simulink model "CopyZeroMain"  (R2023b)
settings: Solver=VariableStepAuto  StartTime=0.0  StopTime=10.0  RelTol=1e-3
values from neighbouring files (symbols this model uses):
  a1 = 40    [FK.m]    (also in IK_Analytical.m = 0.04; IK_MDH.m = 0.04; IK_Position.m = 0.04; IK_Solver.m = 0.04)
  a2 = 275    [FK.m]    (also in IK_Analytical.m = 0.275; IK_MDH.m = 0.275; IK_Position.m = 0.275; IK_Solver.m = 0.275)
  a3 = 25    [FK.m]    (also in IK_Analytical.m = 0.025; IK_MDH.m = 0.025; IK_Position.m = 0.025; IK_Solver.m = 0.025)
  d1 = 342    [FK.m]    (also in IK_Analytical.m = 0.342; IK_MDH.m = 0.342; IK_Position.m = 0.342; IK_Solver.m = 0.342)
  d4 = 280    [FK.m]    (also in IK_Analytical.m = 0.28; IK_MDH.m = 0.28; IK_Position.m = 0.28; IK_Solver.m = 0.28)
  D_H = [ ... (first row only)    [set_mode_parameter.m]
  Ic111 = 0    [set_mode_parameter.m]
  Ic112 = 0    [set_mode_parameter.m]
  Ic113 = 0    [set_mode_parameter.m]
  Ic122 = 0    [set_mode_parameter.m]
  Ic123 = 0    [set_mode_parameter.m]
  Ic133 = 1.3676    [set_mode_parameter.m]
  Ic211 = 8.8194    [set_mode_parameter.m]
  Ic212 = 0    [set_mode_parameter.m]
  Ic213 = 0    [set_mode_parameter.m]
  Ic222 = 6.0549    [set_mode_parameter.m]
  Ic223 = 0    [set_mode_parameter.m]
  Ic233 = 0.9569    [set_mode_parameter.m]
  Ic311 = 0.0332    [set_mode_parameter.m]
  Ic312 = 0    [set_mode_parameter.m]
  Ic313 = 0    [set_mode_parameter.m]
  Ic322 = 1.8442    [set_mode_parameter.m]
  Ic323 = 0    [set_mode_parameter.m]
  Ic333 = 1.0560    (= 1.056)    [set_mode_parameter.m]
  Ic411 = 0.1448    [set_mode_parameter.m]
  Ic412 = 0    [set_mode_parameter.m]
  Ic413 = 0    [set_mode_parameter.m]
  Ic422 = 0.0015    [set_mode_parameter.m]
  Ic423 = 0    [set_mode_parameter.m]
  Ic433 = 0.0822    [set_mode_parameter.m]
  Ic511 = 0    [set_mode_parameter.m]
  Ic512 = 0    [set_mode_parameter.m]
  Ic513 = 0    [set_mode_parameter.m]
  Ic522 = 0.0121    [set_mode_parameter.m]
  Ic523 = 0    [set_mode_parameter.m]
  Ic533 = 0.0299    [set_mode_parameter.m]
  Ic611 = 0.0134    [set_mode_parameter.m]
  Ic612 = 0    [set_mode_parameter.m]
  Ic613 = 0    [set_mode_parameter.m]
  Ic622 = 0    [set_mode_parameter.m]
  Ic623 = 0    [set_mode_parameter.m]
  Ic633 = 0.0051    [set_mode_parameter.m]
  m = (c1*px + s1*py) - dt*(c1*ax + s1*ay) - a1    [IK_6DOF_Robot.m]    (also in IK_MDH.m = pwx_1 - a1; IK_MDH_Robot.m = rho - a1)
  m1 = 0.167    [set_mode_parameter.m]
  m2 = 1    [set_mode_parameter.m]
  m3 = 0.5    [set_mode_parameter.m]
  m4 = 0.333    [set_mode_parameter.m]
  m5 = 0.25    [set_mode_parameter.m]
  m6 = 0.2    [set_mode_parameter.m]
  mc11 = 0    [set_mode_parameter.m]
  mc12 = 0    [set_mode_parameter.m]
  mc13 = 0.2    [set_mode_parameter.m]
  mc21 = 0.1291    [set_mode_parameter.m]
  mc22 = 0    [set_mode_parameter.m]
  mc23 = 3.3117    [set_mode_parameter.m]
  mc31 = 1.6484    [set_mode_parameter.m]
  mc32 = 0    [set_mode_parameter.m]
  mc33 = 0.8748    [set_mode_parameter.m]
  mc41 = 0.3200    (= 0.32)    [set_mode_parameter.m]
  mc42 = 0.2324    [set_mode_parameter.m]
  mc43 = 0.7083    [set_mode_parameter.m]
  mc51 = 0.4574    [set_mode_parameter.m]
  mc52 = 0    [set_mode_parameter.m]
  mc53 = 0.6427    [set_mode_parameter.m]
  mc61 = 0.3200    (= 0.32)    [set_mode_parameter.m]
  mc62 = -0.0513    [set_mode_parameter.m]
  mc63 = 0.6417    [set_mode_parameter.m]
  N = size(waypoints, 2)    [run_trajectory.m]
  s = zc - d(1)    [inverse_kinematics_6dof.m]
  XB4 = SerialLink([L1 L2 L3 L4 L5 L6], 'name', 'XB4')    [Toolbox_Motheds_1.m]
undefined symbols (not defined in the file or in its folder): X, Y, Z
libraries: sm_lib x57, nesl_utility x11
(part 2 of 2)

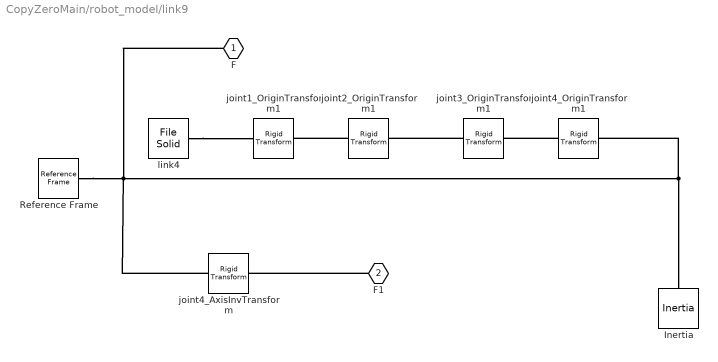
== system CopyZeroMain/robot_model/link9 ==
  Inertia : sm_lib/Body Elements/Inertia  InertiaType=Custom  Mass=m4  MassUnits=kg  CenterOfMass=[mc41 mc42 mc43]  CenterOfMassUnits=m  MomentsOfInertia=[Ic411 Ic422 Ic433]  MomentsOfInertiaUnits=kg*m^2  ProductsOfInertia=[Ic423 Ic413 Ic412]  ProductsOfInertiaUnits=kg*m^2  GraphicType=Marker  MarkerShape=Inertia  MarkerSize=20  GraphicVisPropType=SimpleVisualProperties  GraphicDiffuseColor=[0.5 0.5 0.5]  GraphicSpecularColor=[0.5 0.5 0.5 1.0]  GraphicAmbientColor=[0.15 0.15 0.15 1.0]  GraphicEmissiveColor=[0.0 0.0 0.0 1.0]  GraphicShininess=75  GraphicOpacity=1.0
  Reference Frame : sm_lib/Frames and Transforms/Reference Frame
  joint1_OriginTransform1 : sm_lib/Frames and Transforms/Rigid Transform  TranslationMethod=Cartesian  TranslationStandardOffset=0  TranslationStandardOffsetUnits=m  TranslationStandardAxis=+Z  TranslationCartesianOffset=[0 0 d1]  TranslationCartesianOffsetUnits=m  TranslationROffset=0  TranslationROffsetUnits=m  TranslationZOffset=0  TranslationZOffsetUnits=m  TranslationThetaOffset=0  TranslationThetaOffsetUnits=deg  RotationMethod=RotationSequence  RotationAngleUnits=deg  RotationStandardAxis=+Z  RotationAngle=0.0  RotationArbitraryAxis=[0 0 1]  FollAlignAxisA=+X  BaseAlignAxisA=+Y  FollAlignAxisB=+Y  BaseAlignAxisB=+Z  RotationSequenceAxes=BaseAxes  RotationSequence=XYZ  RotationSequenceAngles=[0 0 0]  RotationSequenceAnglesUnits=rad  RotationMatrix=[1 0 0; 0 1 0; 0 0 1]  Quaternion=[1 0 0 0]
  joint2_OriginTransform1 : sm_lib/Frames and Transforms/Rigid Transform  TranslationMethod=Cartesian  TranslationStandardOffset=0  TranslationStandardOffsetUnits=m  TranslationStandardAxis=+Z  TranslationCartesianOffset=[a1 0 0]  TranslationCartesianOffsetUnits=m  TranslationROffset=0  TranslationROffsetUnits=m  TranslationZOffset=0  TranslationZOffsetUnits=m  TranslationThetaOffset=0  TranslationThetaOffsetUnits=deg  RotationMethod=RotationSequence  RotationAngleUnits=deg  RotationStandardAxis=+Z  RotationAngle=0.0  RotationArbitraryAxis=[0 0 1]  FollAlignAxisA=+X  BaseAlignAxisA=+Y  FollAlignAxisB=+Y  BaseAlignAxisB=+Z  RotationSequenceAxes=FollowerAxes  RotationSequence=XYZ  RotationSequenceAngles=[-pi/2 0 -pi/2]  RotationSequenceAnglesUnits=rad  RotationMatrix=[1 0 0; 0 1 0; 0 0 1]  Quaternion=[1 0 0 0]
  joint3_OriginTransform1 : sm_lib/Frames and Transforms/Rigid Transform  TranslationMethod=Cartesian  TranslationStandardOffset=0  TranslationStandardOffsetUnits=m  TranslationStandardAxis=+Z  TranslationCartesianOffset=[a2 0 0]  TranslationCartesianOffsetUnits=m  TranslationROffset=0  TranslationROffsetUnits=m  TranslationZOffset=0  TranslationZOffsetUnits=m  TranslationThetaOffset=0  TranslationThetaOffsetUnits=deg  RotationMethod=RotationSequence  RotationAngleUnits=deg  RotationStandardAxis=+Z  RotationAngle=0.0  RotationArbitraryAxis=[0 0 1]  FollAlignAxisA=+X  BaseAlignAxisA=+Y  FollAlignAxisB=+Y  BaseAlignAxisB=+Z  RotationSequenceAxes=FollowerAxes  RotationSequence=XYZ  RotationSequenceAngles=[0 0 0]  RotationSequenceAnglesUnits=rad  RotationMatrix=[1 0 0; 0 1 0; 0 0 1]  Quaternion=[1 0 0 0]
  joint4_AxisInvTransform : sm_lib/Frames and Transforms/Rigid Transform  TranslationMethod=Cartesian  TranslationStandardOffset=0  TranslationStandardOffsetUnits=m  TranslationStandardAxis=+Z  TranslationCartesianOffset=[0 0 0]  TranslationCartesianOffsetUnits=m  TranslationROffset=0  TranslationROffsetUnits=m  TranslationZOffset=0  TranslationZOffsetUnits=m  TranslationThetaOffset=0  TranslationThetaOffsetUnits=deg  RotationMethod=RotationSequence  RotationAngleUnits=rad  RotationStandardAxis=+Z  RotationAngle=1.570796  RotationArbitraryAxis=[0 1 0]  FollAlignAxisA=+X  BaseAlignAxisA=+Y  FollAlignAxisB=+Y  BaseAlignAxisB=+Z  RotationSequenceAxes=FollowerAxes  RotationSequence=XYZ  RotationSequenceAngles=[pi/2 0 0]  RotationSequenceAnglesUnits=rad  RotationMatrix=[1 0 0; 0 1 0; 0 0 1]  Quaternion=[1 0 0 0]
  joint4_OriginTransform1 : sm_lib/Frames and Transforms/Rigid Transform  TranslationMethod=Cartesian  TranslationStandardOffset=0  TranslationStandardOffsetUnits=m  TranslationStandardAxis=+Z  TranslationCartesianOffset=[a3 d4 0]  TranslationCartesianOffsetUnits=m  TranslationROffset=0  TranslationROffsetUnits=m  TranslationZOffset=0  TranslationZOffsetUnits=m  TranslationThetaOffset=0  TranslationThetaOffsetUnits=deg  RotationMethod=RotationSequence  RotationAngleUnits=deg  RotationStandardAxis=+Z  RotationAngle=0.0  RotationArbitraryAxis=[0 0 1]  FollAlignAxisA=+X  BaseAlignAxisA=+Y  FollAlignAxisB=+Y  BaseAlignAxisB=+Z  RotationSequenceAxes=FollowerAxes  RotationSequence=XYZ  RotationSequenceAngles=[-pi/2 0 0]  RotationSequenceAnglesUnits=rad  RotationMatrix=[1 0 0; 0 1 0; 0 0 1]  Quaternion=[1 0 0 0]
  link4 : sm_lib/Body Elements/File Solid  ExtGeomFileName=/home/jiehuang/Documents/Custom-Robot/Matlab_Study/Matlab2023Project/IntroductionBook/程序/XB4模型/XB4-4.STL  UnitType=Custom  ExtGeomFileUnits=mm  StepReaderType=HEX  ExportConvexHullGeometry=off  InertiaType=Custom  Mass=0  MassUnits=kg  CenterOfMass=[0 0 0]  CenterOfMassUnits=m  MomentsOfInertia=[0 0 0]  MomentsOfInertiaUnits=kg*m^2  ProductsOfInertia=[0 0 0]  ProductsOfInertiaUnits=kg*m^2  BasedOnType=Density  Density=1000  DensityUnits=kg/(m^3)  DoExposeReferenceFrame=on  SerializedFrames=<Frames/>  GraphicType=FromGeometry  MarkerShape=Sphere  MarkerSize=10  GraphicVisPropType=SimpleVisualProperties  GraphicDiffuseColor=[0.5 0.5 0.5]  GraphicSpecularColor=[0.5 0.5 0.5 1.0]  GraphicAmbientColor=[0.15 0.15 0.15 1.0]  GraphicEmissiveColor=[0.0 0.0 0.0 1.0]  GraphicShininess=75  GraphicOpacity=1.0
  F : PMIOPort  Side=Left
  F1 : PMIOPort  Port=2  Side=Right
  connections:
  Reference Frame/RConn1 -- Inertia/RConn1 -- joint4_OriginTransform1/RConn1 -- F/RConn1 -- joint4_AxisInvTransform/LConn1
  F1/RConn1 -- joint4_AxisInvTransform/RConn1
  joint4_OriginTransform1/LConn1 -- joint3_OriginTransform1/RConn1
  joint3_OriginTransform1/LConn1 -- joint2_OriginTransform1/RConn1
  joint2_OriginTransform1/LConn1 -- joint1_OriginTransform1/RConn1
  link4/RConn1 -- joint1_OriginTransform1/LConn1

== matlab function CopyZeroMain/MATLAB Function1 ==
  data: thetas input; theta output; index input
function theta = theta_selection(thetas, index)

theta = thetas(index, :);

== matlab function CopyZeroMain/inv_kinematic/MATLAB Function13 ==
  data: joint_thetas input; thetas_ret output
function thetas_ret = joint_rad2deg(joint_thetas)
thetas_ret = joint_thetas;
for i = 1:4
    for j = 1:6
        thetas_ret(i,j) = rad2deg(thetas_ret(i,j));
    end
end

== matlab function CopyZeroMain/inv_kinematic/MATLAB Function1 ==
  data: T_target input; joint_thetas_ret output; joint_thetas input; D_H input
function joint_thetas_ret  = get_theta2(T_target, joint_thetas, D_H)
joint_thetas_ret = zeros(4,6);
joint_thetas_ret(1,:) = joint_thetas(1,:);
joint_thetas_ret(2,:) = joint_thetas(1,:);
joint_thetas_ret(3,:) = joint_thetas(2,:);
joint_thetas_ret(4,:) = joint_thetas(2,:);
joint_thetas_ret(1,2) = get_theta2_1(T_target, joint_thetas_ret(1,3), D_H);
joint_thetas_ret(2,2) = get_theta2_2(T_target, joint_thetas_ret(2,3), D_H);
joint_thetas_ret(3,2) = get_theta2_1(T_target, joint_thetas_ret(3,3), D_H);
joint_thetas_ret(4,2) = get_theta2_2(T_target, joint_thetas_ret(4,3), D_H);
end

function theta2_1 = get_theta2_1(T_target, theta3, D_H)
a_cow = D_H(:, 1);
d_cow = D_H(:, 3);
a2 = a_cow(3);
a3 = a_cow(4);
d4 = d_cow(4);
pz = T_target(3,4);
u1_theta2 = -(a2 + (a2^2 + 2*cos(theta3)*a2*a3 - 2*sin(theta3)*a2*d4 + a3^2 + d4^2 - pz^2)^(1/2) + a3*cos(theta3) - d4*sin(theta3))/(d4*cos(theta3) - pz + a3*sin(theta3));
theta2_1 = atan(u1_theta2)*2;
end

function theta2_2 = get_theta2_2(T_target, theta3, D_H)
a_cow = D_H(:, 1);
d_cow = D_H(:, 3);
a2 = a_cow(3);
a3 = a_cow(4);
d4 = d_cow(4);
pz = T_target(3,4);
u2_theta2 = -(a2 - (a2^2 + 2*cos(theta3)*a2*a3 - 2*sin(theta3)*a2*d4 + a3^2 + d4^2 - pz^2)^(1/2) + a3*cos(theta3) - d4*sin(theta3))/(d4*cos(theta3) - pz + a3*sin(theta3));
theta2_2 = atan(u2_theta2)*2;
end

== matlab function CopyZeroMain/inv_kinematic/MATLAB Function ==
  data: T_target input; joint_theatas_ret output; D_H input
function joint_theatas_ret  = get_theta3(T_target, D_H)
a_cow = D_H(:, 1);
d_cow = D_H(:, 3);
a2 = a_cow(3);
a3 = a_cow(4);
d4 = d_cow(4);
px = T_target(1,4);
py = T_target(2,4);
pz = T_target(3,4);
joint_theatas_ret = zeros(2,6);

u1_theta3 = -(2*a2*d4 + (- a2^4 + 2*a2^2*a3^2 + 2*a2^2*d4^2 + 2*a2^2*px^2 + 2*a2^2*py^2 + 2*a2^2*pz^2 - a3^4 - 2*a3^2*d4^2 + 2*a3^2*px^2 + 2*a3^2*py^2 + 2*a3^2*pz^2 - d4^4 + 2*d4^2*px^2 + 2*d4^2*py^2 + 2*d4^2*pz^2 - px^4 - 2*px^2*py^2 - 2*px^2*pz^2 - py^4 - 2*py^2*pz^2 - pz^4)^(1/2))/(- a2^2 + 2*a2*a3 - a3^2 - d4^2 + px^2 + py^2 + pz^2);
u2_theta3 = -(2*a2*d4 - (- a2^4 + 2*a2^2*a3^2 + 2*a2^2*d4^2 + 2*a2^2*px^2 + 2*a2^2*py^2 + 2*a2^2*pz^2 - a3^4 - 2*a3^2*d4^2 + 2*a3^2*px^2 + 2*a3^2*py^2 + 2*a3^2*pz^2 - d4^4 + 2*d4^2*px^2 + 2*d4^2*py^2 + 2*d4^2*pz^2 - px^4 - 2*px^2*py^2 - 2*px^2*pz^2 - py^4 - 2*py^2*pz^2 - pz^4)^(1/2))/(- a2^2 + 2*a2*a3 - a3^2 - d4^2 + px^2 + py^2 + pz^2);
theta3_1 = atan(u1_theta3)*2;
theta3_2 = atan(u2_theta3)*2;
joint_theatas_ret(1, 3) = theta3_1;
joint_theatas_ret(2, 3) = theta3_2;
end

== matlab function CopyZeroMain/inv_kinematic/MATLAB Function2 ==
  data: T_target input; joint_thetas output; joint_thetas input; D_H input
function joint_thetas  = get_theta1(T_target, joint_thetas, D_H)
joint_thetas(1,1) = get_theta1_(T_target, joint_thetas(1,:), D_H);
joint_thetas(2,1) = get_theta1_(T_target, joint_thetas(2,:), D_H);
joint_thetas(3,1) = get_theta1_(T_target, joint_thetas(3,:), D_H);
joint_thetas(4,1) = get_theta1_(T_target, joint_thetas(4,:), D_H);
end

function theta1_1 = get_theta1_(T_target, thetas, D_H)
a_cow = D_H(:, 1);
d_cow = D_H(:, 3);
a2 = a_cow(3);
a3 = a_cow(4);
d4 = d_cow(4);
px = T_target(1,4);
py = T_target(2,4);
pz = T_target(3,4);

theta2 = thetas(2);
theta3 = thetas(3);

v1 = (cos(theta2)*(a2 + a3*cos(theta3) - d4*sin(theta3)) + sin(theta2)*(d4*cos(theta3) + a3*sin(theta3)));
v2 = -px/v1;

% 设置容忍度
tolerance = 1e-4;

u1_theta1 = ((v2+1)/(1-v2))^(1/2);
if abs(py - (2*u1_theta1*v1)/(u1_theta1^2 + 1)) > tolerance
    u1_theta1 = -u1_theta1;
end
theta1_1 = atan(u1_theta1)*2;
end

== matlab function CopyZeroMain/inv_kinematic/MATLAB Function3 ==
  data: T_target input; joint_thetas_ret output; joint_thetas input; D_H input
function joint_thetas_ret  = get_theta5(T_target, joint_thetas, D_H)
joint_thetas_ret = joint_thetas;
for i = 1:4
    joint_thetas_ret(i, 5) = get_theta5_(T_target, joint_thetas_ret(i, :), D_H);
end
end

function theta5 = get_theta5_(T_target, thetas, D_H)
a_cow = D_H(:, 1);
d_cow = D_H(:, 3);
a2 = a_cow(3);
a3 = a_cow(4);
d4 = d_cow(4);
px = T_target(1,4);
py = T_target(2,4);
pz = T_target(3,4);
nx = T_target(1,1);
ny = T_target(2,1);
nz = T_target(3,1);
ox = T_target(1,2);
oy = T_target(2,2);
oz = T_target(3,2);
ax= T_target(1,3);
ay= T_target(2,3);
az= T_target(3,3);
theta2 = thetas(2);
theta3 = thetas(3);
theta1 = thetas(1);

r32 = - (oz*(cos(theta2)*cos(theta3) + sin(theta2)*sin(theta3)))/(cos(theta2)^2*cos(theta3)^2 + cos(theta2)^2*sin(theta3)^2 + cos(theta3)^2*sin(theta2)^2 + sin(theta2)^2*sin(theta3)^2) - (ox*(cos(theta1)*cos(theta2)*sin(theta3) - cos(theta1)*cos(theta3)*sin(theta2)))/(cos(theta1)^2*cos(theta2)^2*cos(theta3)^2 + cos(theta1)^2*cos(theta2)^2*sin(theta3)^2 + cos(theta1)^2*cos(theta3)^2*sin(theta2)^2 + cos(theta1)^2*sin(theta2)^2*sin(theta3)^2 + cos(theta2)^2*cos(theta3)^2*sin(theta1)^2 + cos(theta2)^2*sin(theta1)^2*sin(theta3)^2 + cos(theta3)^2*sin(theta1)^2*sin(theta2)^2 + sin(theta1)^2*sin(theta2)^2*sin(theta3)^2) - (oy*(cos(theta2)*sin(theta1)*sin(theta3) - cos(theta3)*sin(theta1)*sin(theta2)))/(cos(theta1)^2*cos(theta2)^2*cos(theta3)^2 + cos(theta1)^2*cos(theta2)^2*sin(theta3)^2 + cos(theta1)^2*cos(theta3)^2*sin(theta2)^2 + cos(theta1)^2*sin(theta2)^2*sin(theta3)^2 + cos(theta2)^2*cos(theta3)^2*sin(theta1)^2 + cos(theta2)^2*sin(theta1)^2*sin(theta3)^2 + cos(theta3)^2*sin(theta1)^2*sin(theta2)^2 + sin(theta1)^2*sin(theta2)^2*sin(theta3)^2);
r31 = - (nz*(cos(theta2)*cos(theta3) + sin(theta2)*sin(theta3)))/(cos(theta2)^2*cos(theta3)^2 + cos(theta2)^2*sin(theta3)^2 + cos(theta3)^2*sin(theta2)^2 + sin(theta2)^2*sin(theta3)^2) - (nx*(cos(theta1)*cos(theta2)*sin(theta3) - cos(theta1)*cos(theta3)*sin(theta2)))/(cos(theta1)^2*cos(theta2)^2*cos(theta3)^2 + cos(theta1)^2*cos(theta2)^2*sin(theta3)^2 + cos(theta1)^2*cos(theta3)^2*sin(theta2)^2 + cos(theta1)^2*sin(theta2)^2*sin(theta3)^2 + cos(theta2)^2*cos(theta3)^2*sin(theta1)^2 + cos(theta2)^2*sin(theta1)^2*sin(theta3)^2 + cos(theta3)^2*sin(theta1)^2*sin(theta2)^2 + sin(theta1)^2*sin(theta2)^2*sin(theta3)^2) - (ny*(cos(theta2)*sin(theta1)*sin(theta3) - cos(theta3)*sin(theta1)*sin(theta2)))/(cos(theta1)^2*cos(theta2)^2*cos(theta3)^2 + cos(theta1)^2*cos(theta2)^2*sin(theta3)^2 + cos(theta1)^2*cos(theta3)^2*sin(theta2)^2 + cos(theta1)^2*sin(theta2)^2*sin(theta3)^2 + cos(theta2)^2*cos(theta3)^2*sin(theta1)^2 + cos(theta2)^2*sin(theta1)^2*sin(theta3)^2 + cos(theta3)^2*sin(theta1)^2*sin(theta2)^2 + sin(theta1)^2*sin(theta2)^2*sin(theta3)^2);
r33 = - (az*(cos(theta2)*cos(theta3) + sin(theta2)*sin(theta3)))/(cos(theta2)^2*cos(theta3)^2 + cos(theta2)^2*sin(theta3)^2 + cos(theta3)^2*sin(theta2)^2 + sin(theta2)^2*sin(theta3)^2) - (ax*(cos(theta1)*cos(theta2)*sin(theta3) - cos(theta1)*cos(theta3)*sin(theta2)))/(cos(theta1)^2*cos(theta2)^2*cos(theta3)^2 + cos(theta1)^2*cos(theta2)^2*sin(theta3)^2 + cos(theta1)^2*cos(theta3)^2*sin(theta2)^2 + cos(theta1)^2*sin(theta2)^2*sin(theta3)^2 + cos(theta2)^2*cos(theta3)^2*sin(theta1)^2 + cos(theta2)^2*sin(theta1)^2*sin(theta3)^2 + cos(theta3)^2*sin(theta1)^2*sin(theta2)^2 + sin(theta1)^2*sin(theta2)^2*sin(theta3)^2) - (ay*(cos(theta2)*sin(theta1)*sin(theta3) - cos(theta3)*sin(theta1)*sin(theta2)))/(cos(theta1)^2*cos(theta2)^2*cos(theta3)^2 + cos(theta1)^2*cos(theta2)^2*sin(theta3)^2 + cos(theta1)^2*cos(theta3)^2*sin(theta2)^2 + cos(theta1)^2*sin(theta2)^2*sin(theta3)^2 + cos(theta2)^2*cos(theta3)^2*sin(theta1)^2 + cos(theta2)^2*sin(theta1)^2*sin(theta3)^2 + cos(theta3)^2*sin(theta1)^2*sin(theta2)^2 + sin(theta1)^2*sin(theta2)^2*sin(theta3)^2);
theta5 = atan2(sqrt(r32^2 + r31^2), r33);
theta5 = -theta5 + pi;
end

== matlab function CopyZeroMain/inv_kinematic/MATLAB Function4 ==
  data: T_target input; joint_thetas_ret output; joint_thetas input; D_H input
function joint_thetas_ret  = get_theta4(T_target, joint_thetas, D_H)
joint_thetas_ret = joint_thetas;
for i = 1:4
    joint_thetas_ret(i, 4) = get_theta4_(T_target, joint_thetas_ret(i, :), D_H);
end
end

function theta4_value = get_theta4_(T_target, thetas, D_H)
% deg_theta5_zyz = rad2deg(-thetas(5) + pi);
% if deg_theta5_zyz == 0 || deg_theta5_zyz == 180
%     theta4_value = 0;
%     return;
% end
a_cow = D_H(:, 1);
d_cow = D_H(:, 3);
a2 = a_cow(3);
a3 = a_cow(4);
d4 = d_cow(4);
px = T_target(1,4);
py = T_target(2,4);
pz = T_target(3,4);
nx = T_target(1,1);
ny = T_target(2,1);
nz = T_target(3,1);
ox = T_target(1,2);
oy = T_target(2,2);
oz = T_target(3,2);
ax= T_target(1,3);
ay= T_target(2,3);
az= T_target(3,3);
theta2 = thetas(2);
theta3 = thetas(3);
theta1 = thetas(1);
theta4 = 0; % 这里特殊，用于坐标系对齐
r23 = -(ax*cos(theta1)*cos(theta2)*cos(theta3)*sin(theta4) - ax*cos(theta4)*sin(theta1)*sin(theta2)^2*sin(theta3)^2 + ay*cos(theta2)*cos(theta3)*sin(theta1)*sin(theta4) + ax*cos(theta1)*sin(theta2)*sin(theta3)*sin(theta4) + ay*sin(theta1)*sin(theta2)*sin(theta3)*sin(theta4) - az*cos(theta1)^2*cos(theta2)*sin(theta3)*sin(theta4) + az*cos(theta1)^2*cos(theta3)*sin(theta2)*sin(theta4) - az*cos(theta2)*sin(theta1)^2*sin(theta3)*sin(theta4) + az*cos(theta3)*sin(theta1)^2*sin(theta2)*sin(theta4) + ay*cos(theta1)*cos(theta2)^2*cos(theta3)^2*cos(theta4) - ax*cos(theta2)^2*cos(theta3)^2*cos(theta4)*sin(theta1) + ay*cos(theta1)*cos(theta2)^2*cos(theta4)*sin(theta3)^2 + ay*cos(theta1)*cos(theta3)^2*cos(theta4)*sin(theta2)^2 - ax*cos(theta2)^2*cos(theta4)*sin(theta1)*sin(theta3)^2 - ax*cos(theta3)^2*cos(theta4)*sin(theta1)*sin(theta2)^2 + ay*cos(theta1)*cos(theta4)*sin(theta2)^2*sin(theta3)^2)/((cos(theta1)^2*cos(theta4)^2 + cos(theta1)^2*sin(theta4)^2 + cos(theta4)^2*sin(theta1)^2 + sin(theta1)^2*sin(theta4)^2)*(cos(theta2)^2*cos(theta3)^2 + cos(theta2)^2*sin(theta3)^2 + cos(theta3)^2*sin(theta2)^2 + sin(theta2)^2*sin(theta3)^2));
r13 = (-az*cos(theta4)*cos(theta1)^2*cos(theta2)*sin(theta3) + az*cos(theta4)*cos(theta1)^2*cos(theta3)*sin(theta2) - ay*sin(theta4)*cos(theta1)*cos(theta2)^2*cos(theta3)^2 - ay*sin(theta4)*cos(theta1)*cos(theta2)^2*sin(theta3)^2 + ax*cos(theta4)*cos(theta1)*cos(theta2)*cos(theta3) - ay*sin(theta4)*cos(theta1)*cos(theta3)^2*sin(theta2)^2 - ay*sin(theta4)*cos(theta1)*sin(theta2)^2*sin(theta3)^2 + ax*cos(theta4)*cos(theta1)*sin(theta2)*sin(theta3) + ax*sin(theta4)*cos(theta2)^2*cos(theta3)^2*sin(theta1) + ax*sin(theta4)*cos(theta2)^2*sin(theta1)*sin(theta3)^2 + ay*cos(theta4)*cos(theta2)*cos(theta3)*sin(theta1) - az*cos(theta4)*cos(theta2)*sin(theta1)^2*sin(theta3) + ax*sin(theta4)*cos(theta3)^2*sin(theta1)*sin(theta2)^2 + az*cos(theta4)*cos(theta3)*sin(theta1)^2*sin(theta2) + ax*sin(theta4)*sin(theta1)*sin(theta2)^2*sin(theta3)^2 + ay*cos(theta4)*sin(theta1)*sin(theta2)*sin(theta3))/((cos(theta1)^2 + sin(theta1)^2)*(cos(theta4)^2 + sin(theta4)^2)*(cos(theta2)^2*cos(theta3)^2 + cos(theta2)^2*sin(theta3)^2 + cos(theta3)^2*sin(theta2)^2 + sin(theta2)^2*sin(theta3)^2));
theta4_value = atan2(r23, r13);
end

== matlab function CopyZeroMain/inv_kinematic/MATLAB Function5 ==
  data: T_target input; joint_thetas_ret output; joint_thetas input; D_H input
function joint_thetas_ret  = get_theta6(T_target, joint_thetas, D_H)
joint_thetas_ret = joint_thetas;
for i = 1:4
    joint_thetas_ret(i, 6) = get_theta6_(T_target, joint_thetas_ret(i, :), D_H);
end
end

function theta6_value = get_theta6_(T_target, thetas, D_H)
a_cow = D_H(:, 1);
d_cow = D_H(:, 3);
a2 = a_cow(3);
a3 = a_cow(4);
d4 = d_cow(4);
px = T_target(1,4);
py = T_target(2,4);
pz = T_target(3,4);
nx = T_target(1,1);
ny = T_target(2,1);
nz = T_target(3,1);
ox = T_target(1,2);
oy = T_target(2,2);
oz = T_target(3,2);
ax= T_target(1,3);
ay= T_target(2,3);
az= T_target(3,3);
theta2 = thetas(2);
theta3 = thetas(3);
theta1 = thetas(1);
theta4 = 0;
% deg_theta5_zyz = rad2deg(-thetas(5) + pi);
% if deg_theta5_zyz == 0 || deg_theta5_zyz == 180
%     r12 = (ox*(sin(theta1)*sin(theta4)*cos(theta2)^2*cos(theta3)^2 + sin(theta1)*sin(theta4)*cos(theta2)^2*sin(theta3)^2 + cos(theta1)*cos(theta4)*cos(theta2)*cos(theta3) + sin(theta1)*sin(theta4)*cos(theta3)^2*sin(theta2)^2 + sin(theta1)*sin(theta4)*sin(theta2)^2*sin(theta3)^2 + cos(theta1)*cos(theta4)*sin(theta2)*sin(theta3)))/(cos(theta1)^2*cos(theta2)^2*cos(theta3)^2*cos(theta4)^2 + cos(theta1)^2*cos(theta2)^2*cos(theta3)^2*sin(theta4)^2 + cos(theta1)^2*cos(theta2)^2*cos(theta4)^2*sin(theta3)^2 + cos(theta1)^2*cos(theta2)^2*sin(theta3)^2*sin(theta4)^2 + cos(theta1)^2*cos(theta3)^2*cos(theta4)^2*sin(theta2)^2 + cos(theta1)^2*cos(theta3)^2*sin(theta2)^2*sin(theta4)^2 + cos(theta1)^2*cos(theta4)^2*sin(theta2)^2*sin(theta3)^2 + cos(theta1)^2*sin(theta2)^2*sin(theta3)^2*sin(theta4)^2 + cos(theta2)^2*cos(theta3)^2*cos(theta4)^2*sin(theta1)^2 + cos(theta2)^2*cos(theta3)^2*sin(theta1)^2*sin(theta4)^2 + cos(theta2)^2*cos(theta4)^2*sin(theta1)^2*sin(theta3)^2 + cos(theta2)^2*sin(theta1)^2*sin(theta3)^2*sin(theta4)^2 + cos(theta3)^2*cos(theta4)^2*sin(theta1)^2*sin(theta2)^2 + cos(theta3)^2*sin(theta1)^2*sin(theta2)^2*sin(theta4)^2 + cos(theta4)^2*sin(theta1)^2*sin(theta2)^2*sin(theta3)^2 + sin(theta1)^2*sin(theta2)^2*sin(theta3)^2*sin(theta4)^2) - (oz*(cos(theta2)*cos(theta4)*sin(theta3) - cos(theta3)*cos(theta4)*sin(theta2)))/(cos(theta2)^2*cos(theta3)^2*cos(theta4)^2 + cos(theta2)^2*cos(theta3)^2*sin(theta4)^2 + cos(theta2)^2*cos(theta4)^2*sin(theta3)^2 + cos(theta2)^2*sin(theta3)^2*sin(theta4)^2 + cos(theta3)^2*cos(theta4)^2*sin(theta2)^2 + cos(theta3)^2*sin(theta2)^2*sin(theta4)^2 + cos(theta4)^2*sin(theta2)^2*sin(theta3)^2 + sin(theta2)^2*sin(theta3)^2*sin(theta4)^2) - (oy*(cos(theta1)*sin(theta4)*cos(theta2)^2*cos(theta3)^2 + cos(theta1)*sin(theta4)*cos(theta2)^2*sin(theta3)^2 - cos(theta4)*sin(theta1)*cos(theta2)*cos(theta3) + cos(theta1)*sin(theta4)*cos(theta3)^2*sin(theta2)^2 + cos(theta1)*sin(theta4)*sin(theta2)^2*sin(theta3)^2 - cos(theta4)*sin(theta1)*sin(theta2)*sin(theta3)))/(cos(theta1)^2*cos(theta2)^2*cos(theta3)^2*cos(theta4)^2 + cos(theta1)^2*cos(theta2)^2*cos(theta3)^2*sin(theta4)^2 + cos(theta1)^2*cos(theta2)^2*cos(theta4)^2*sin(theta3)^2 + cos(theta1)^2*cos(theta2)^2*sin(theta3)^2*sin(theta4)^2 + cos(theta1)^2*cos(theta3)^2*cos(theta4)^2*sin(theta2)^2 + cos(theta1)^2*cos(theta3)^2*sin(theta2)^2*sin(theta4)^2 + cos(theta1)^2*cos(theta4)^2*sin(theta2)^2*sin(theta3)^2 + cos(theta1)^2*sin(theta2)^2*sin(theta3)^2*sin(theta4)^2 + cos(theta2)^2*cos(theta3)^2*cos(theta4)^2*sin(theta1)^2 + cos(theta2)^2*cos(theta3)^2*sin(theta1)^2*sin(theta4)^2 + cos(theta2)^2*cos(theta4)^2*sin(theta1)^2*sin(theta3)^2 + cos(theta2)^2*sin(theta1)^2*sin(theta3)^2*sin(theta4)^2 + cos(theta3)^2*cos(theta4)^2*sin(theta1)^2*sin(theta2)^2 + cos(theta3)^2*sin(theta1)^2*sin(theta2)^2*sin(theta4)^2 + cos(theta4)^2*sin(theta1)^2*sin(theta2)^2*sin(theta3)^2 + sin(theta1)^2*sin(theta2)^2*sin(theta3)^2*sin(theta4)^2);
%     r11 = (nx*(sin(theta1)*sin(theta4)*cos(theta2)^2*cos(theta3)^2 + sin(theta1)*sin(theta4)*cos(theta2)^2*sin(theta3)^2 + cos(theta1)*cos(theta4)*cos(theta2)*cos(theta3) + sin(theta1)*sin(theta4)*cos(theta3)^2*sin(theta2)^2 + sin(theta1)*sin(theta4)*sin(theta2)^2*sin(theta3)^2 + cos(theta1)*cos(theta4)*sin(theta2)*sin(theta3)))/(cos(theta1)^2*cos(theta2)^2*cos(theta3)^2*cos(theta4)^2 + cos(theta1)^2*cos(theta2)^2*cos(theta3)^2*sin(theta4)^2 + cos(theta1)^2*cos(theta2)^2*cos(theta4)^2*sin(theta3)^2 + cos(theta1)^2*cos(theta2)^2*sin(theta3)^2*sin(theta4)^2 + cos(theta1)^2*cos(theta3)^2*cos(theta4)^2*sin(theta2)^2 + cos(theta1)^2*cos(theta3)^2*sin(theta2)^2*sin(theta4)^2 + cos(theta1)^2*cos(theta4)^2*sin(theta2)^2*sin(theta3)^2 + cos(theta1)^2*sin(theta2)^2*sin(theta3)^2*sin(theta4)^2 + cos(theta2)^2*cos(theta3)^2*cos(theta4)^2*sin(theta1)^2 + cos(theta2)^2*cos(theta3)^2*sin(theta1)^2*sin(theta4)^2 + cos(theta2)^2*cos(theta4)^2*sin(theta1)^2*sin(theta3)^2 + cos(theta2)^2*sin(theta1)^2*sin(theta3)^2*sin(theta4)^2 + cos(theta3)^2*cos(theta4)^2*sin(theta1)^2*sin(theta2)^2 + cos(theta3)^2*sin(theta1)^2*sin(theta2)^2*sin(theta4)^2 + cos(theta4)^2*sin(theta1)^2*sin(theta2)^2*sin(theta3)^2 + sin(theta1)^2*sin(theta2)^2*sin(theta3)^2*sin(theta4)^2) - (nz*(cos(theta2)*cos(theta4)*sin(theta3) - cos(theta3)*cos(theta4)*sin(theta2)))/(cos(theta2)^2*cos(theta3)^2*cos(theta4)^2 + cos(theta2)^2*cos(theta3)^2*sin(theta4)^2 + cos(theta2)^2*cos(theta4)^2*sin(theta3)^2 + cos(theta2)^2*sin(theta3)^2*sin(theta4)^2 + cos(theta3)^2*cos(theta4)^2*sin(theta2)^2 + cos(theta3)^2*sin(theta2)^2*sin(theta4)^2 + cos(theta4)^2*sin(theta2)^2*sin(theta3)^2 + sin(theta2)^2*sin(theta3)^2*sin(theta4)^2) - (ny*(cos(theta1)*sin(theta4)*cos(theta2)^2*cos(theta3)^2 + cos(theta1)*sin(theta4)*cos(theta2)^2*sin(theta3)^2 - cos(theta4)*sin(theta1)*cos(theta2)*cos(theta3) + cos(theta1)*sin(theta4)*cos(theta3)^2*sin(theta2)^2 + cos(theta1)*sin(theta4)*sin(theta2)^2*sin(theta3)^2 - cos(theta4)*sin(theta1)*sin(theta2)*sin(theta3)))/(cos(theta1)^2*cos(theta2)^2*cos(theta3)^2*cos(theta4)^2 + cos(theta1)^2*cos(theta2)^2*cos(theta3)^2*sin(theta4)^2 + cos(theta1)^2*cos(theta2)^2*cos(theta4)^2*sin(theta3)^2 + cos(theta1)^2*cos(theta2)^2*sin(theta3)^2*sin(theta4)^2 + cos(theta1)^2*cos(theta3)^2*cos(theta4)^2*sin(theta2)^2 + cos(theta1)^2*cos(theta3)^2*sin(theta2)^2*sin(theta4)^2 + cos(theta1)^2*cos(theta4)^2*sin(theta2)^2*sin(theta3)^2 + cos(theta1)^2*sin(theta2)^2*sin(theta3)^2*sin(theta4)^2 + cos(theta2)^2*cos(theta3)^2*cos(theta4)^2*sin(theta1)^2 + cos(theta2)^2*cos(theta3)^2*sin(theta1)^2*sin(theta4)^2 + cos(theta2)^2*cos(theta4)^2*sin(theta1)^2*sin(theta3)^2 + cos(theta2)^2*sin(theta1)^2*sin(theta3)^2*sin(theta4)^2 + cos(theta3)^2*cos(theta4)^2*sin(theta1)^2*sin(theta2)^2 + cos(theta3)^2*sin(theta1)^2*sin(theta2)^2*sin(theta4)^2 + cos(theta4)^2*sin(theta1)^2*sin(theta2)^2*sin(theta3)^2 + sin(theta1)^2*sin(theta2)^2*sin(theta3)^2*sin(theta4)^2);
%     theta6_value = atan2(-r12, r11);
%     theta6_value = theta6_value - pi;
%     return;
% end

r32 = - (oz*(cos(theta2)*cos(theta3) + sin(theta2)*sin(theta3)))/(cos(theta2)^2*cos(theta3)^2 + cos(theta2)^2*sin(theta3)^2 + cos(theta3)^2*sin(theta2)^2 + sin(theta2)^2*sin(theta3)^2) - (ox*(cos(theta1)*cos(theta2)*sin(theta3) - cos(theta1)*cos(theta3)*sin(theta2)))/(cos(theta1)^2*cos(theta2)^2*cos(theta3)^2 + cos(theta1)^2*cos(theta2)^2*sin(theta3)^2 + cos(theta1)^2*cos(theta3)^2*sin(theta2)^2 + cos(theta1)^2*sin(theta2)^2*sin(theta3)^2 + cos(theta2)^2*cos(theta3)^2*sin(theta1)^2 + cos(theta2)^2*sin(theta1)^2*sin(theta3)^2 + cos(theta3)^2*sin(theta1)^2*sin(theta2)^2 + sin(theta1)^2*sin(theta2)^2*sin(theta3)^2) - (oy*(cos(theta2)*sin(theta1)*sin(theta3) - cos(theta3)*sin(theta1)*sin(theta2)))/(cos(theta1)^2*cos(theta2)^2*cos(theta3)^2 + cos(theta1)^2*cos(theta2)^2*sin(theta3)^2 + cos(theta1)^2*cos(theta3)^2*sin(theta2)^2 + cos(theta1)^2*sin(theta2)^2*sin(theta3)^2 + cos(theta2)^2*cos(theta3)^2*sin(theta1)^2 + cos(theta2)^2*sin(theta1)^2*sin(theta3)^2 + cos(theta3)^2*sin(theta1)^2*sin(theta2)^2 + sin(theta1)^2*sin(theta2)^2*sin(theta3)^2);
r31 = - (nz*(cos(theta2)*cos(theta3) + sin(theta2)*sin(theta3)))/(cos(theta2)^2*cos(theta3)^2 + cos(theta2)^2*sin(theta3)^2 + cos(theta3)^2*sin(theta2)^2 + sin(theta2)^2*sin(theta3)^2) - (nx*(cos(theta1)*cos(theta2)*sin(theta3) - cos(theta1)*cos(theta3)*sin(theta2)))/(cos(theta1)^2*cos(theta2)^2*cos(theta3)^2 + cos(theta1)^2*cos(theta2)^2*sin(theta3)^2 + cos(theta1)^2*cos(theta3)^2*sin(theta2)^2 + cos(theta1)^2*sin(theta2)^2*sin(theta3)^2 + cos(theta2)^2*cos(theta3)^2*sin(theta1)^2 + cos(theta2)^2*sin(theta1)^2*sin(theta3)^2 + cos(theta3)^2*sin(theta1)^2*sin(theta2)^2 + sin(theta1)^2*sin(theta2)^2*sin(theta3)^2) - (ny*(cos(theta2)*sin(theta1)*sin(theta3) - cos(theta3)*sin(theta1)*sin(theta2)))/(cos(theta1)^2*cos(theta2)^2*cos(theta3)^2 + cos(theta1)^2*cos(theta2)^2*sin(theta3)^2 + cos(theta1)^2*cos(theta3)^2*sin(theta2)^2 + cos(theta1)^2*sin(theta2)^2*sin(theta3)^2 + cos(theta2)^2*cos(theta3)^2*sin(theta1)^2 + cos(theta2)^2*sin(theta1)^2*sin(theta3)^2 + cos(theta3)^2*sin(theta1)^2*sin(theta2)^2 + sin(theta1)^2*sin(theta2)^2*sin(theta3)^2);
theta6_value = atan2(r32, -r31);
theta6_value = theta6_value - pi;
end

== matlab function CopyZeroMain/inv_kinematic/MATLAB Function6 ==
  data: joint_thetas input; D_H input; theta_ret output; thetas output; theta_diffs output; best_diff_index output
function [theta_ret, thetas, theta_diffs, best_diff_index]  = get_best_joint_theta(joint_thetas, D_H)
% theta_ret: 最优一组的关节相对于初始位置的旋转角度
% thetas: 所有组的关节相对于初始位置的旋转角度
% theta_diffs：所有组的与当前关节角度变化的绝对值总和，即与当前位置的差异，其大小表示需要变化的难度
thetas = joint_thetas;
    theta_diffs = zeros(1,4);
    persistent current_theta
    if isempty(current_theta)
        current_theta = zeros(1,6);
    end

    for i = 1:4
        [theta, theta_diff] = joint_theta_change(thetas(i, :), current_theta, D_H);
        thetas(i, :) = theta;
        theta_diffs(i) = theta_diff;
    end
    [~, best_diff_index] = min(theta_diffs);
    theta_ret = thetas(best_diff_index, :);
    current_theta = theta_ret;
end

function [theta_ret, theta_diff] = joint_theta_change(theta, current_theta, D_H)
    % theta_diff: 与当前关节角度变化的绝对值总和，即与当前位置的差异，其大小表示需要变化的难度
    theta_ret = zeros(1,6);
    theta_diff = 0;
    for i = 1:6
        tmp_theta = mod(theta(i) + 360, 360);
        init_theta = mod(rad2deg(D_H(i, 4)) + 360, 360);
        theta_ret(i) = tmp_theta - init_theta;
        theta_diff = theta_diff + (7 - i) * abs(theta_ret(i) - current_theta(i)); % 与当前位置的差异
    end
end

== matlab function CopyZeroMain/MATLAB Function ==
  data: xyz input; T_target output; rot input
function T_target = T_target_genrate(xyz, rot)
T_target = [rot xyz; 0 0 0 1];

== matlab function CopyZeroMain/kinematics/MATLAB Function ==
  data: D_H input; T0_1 output; T1_2 output; T2_3 output; T3_4 output; T4_5 output; T5_6 output; joints_theata input; T0_6 output
function [T0_1, T1_2, T2_3, T3_4, T4_5, T5_6, T0_6] = get_links_trans(D_H, joints_theata)
% 获得连杆变化矩阵
% D_H: D-H表
% joints_theta: 当前各关节角度 rad
T0_1 = get_link_trans(D_H(1,:), joints_theata(1));
T1_2 = get_link_trans(D_H(2,:), joints_theata(2));
T2_3 = get_link_trans(D_H(3,:), joints_theata(3));
T3_4 = get_link_trans(D_H(4,:), joints_theata(4));
T4_5 = get_link_trans(D_H(5,:), joints_theata(5));
T5_6 = get_link_trans(D_H(6,:), joints_theata(6));
T0_6 = T0_1 * T1_2 * T2_3 * T3_4 * T4_5 * T5_6;
end

function T = get_link_trans(D_H_link, joint_theta)
a = D_H_link(1);
alpha = D_H_link(2);
d = D_H_link(3);
theta = joint_theta;
T = [cos(theta), -sin(theta), 0, a;
    sin(theta)*cos(alpha), cos(theta)*cos(alpha), -sin(alpha), -d*sin(alpha);
    sin(theta)*sin(alpha), cos(theta)*sin(alpha), cos(alpha), d*cos(alpha);
    0, 0, 0, 1];
end
